simulink model "read_acs712"  (R2021b)
settings: Solver=ode1  StartTime=0.0  StopTime=30  FixedStep=0.01  RelTol=1e-3  EnableMultiTasking=on
libraries: arduinolib x3, dspstat3 x1
settings Model: ExtModeTrigDuration=2  Creator=ASUS  LastModifiedBy=ASUS
settings OptimizationCC: EnhancedBackFolding=on  PassReuseOutputArgsAs=Individual arguments  ZeroExternalMemoryAtStartup=off  ZeroInternalMemoryAtStartup=off  MaxStackSize=64  OptimizeBlockOrder=speed  DifferentSizesBufferReuse=on  OptimizationCustomize=off  EfficientTunableParamExpr=on
settings DebuggingCC: ParameterTunabilityLossMsg=error
settings HardwareCC: ProdBitPerInt=16  ProdBitPerPointer=16  ProdBitPerSizeT=16  ProdBitPerPtrDiffT=16  ProdLargestAtomicFloat=None  ProdWordSize=8  ProdHWDeviceType=Atmel->AVR
settings SFSimCC: MATLABDynamicMemAlloc=off
settings RTWCC: Description=Embedded Coder  SystemTargetFile=ert.tlc  HardwareBoard=Arduino Uno  TemplateMakefile=ert_default_tmf  Toolchain=Arduino AVR  BuildConfiguration=Faster Runs
settings CodeAppCC: ForceParamTrailComments=on  IgnoreCustomStorageClasses=off  OperatorAnnotations=on  SimulinkDataObjDesc=on  SFDataObjDesc=on  InsertBlockDesc=on
settings ERTTargetCC: SupportContinuousTime=on  SupportNonInlinedSFcns=on  SupportVariableSizeSignals=on  ExtModeTransport=3  ExtModeStaticAlloc=on  ExtModeStaticAllocSize=250  ExtModeMexFile=ext_xcp  ExtModeIntrfLevel=Level2 - Open

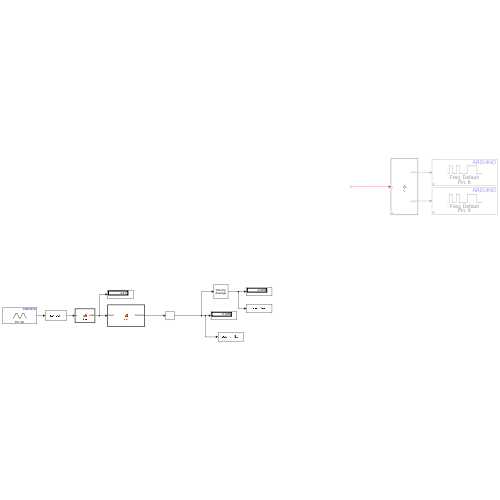
[thumbnail: Simulink's stored preview of the top-level diagram]
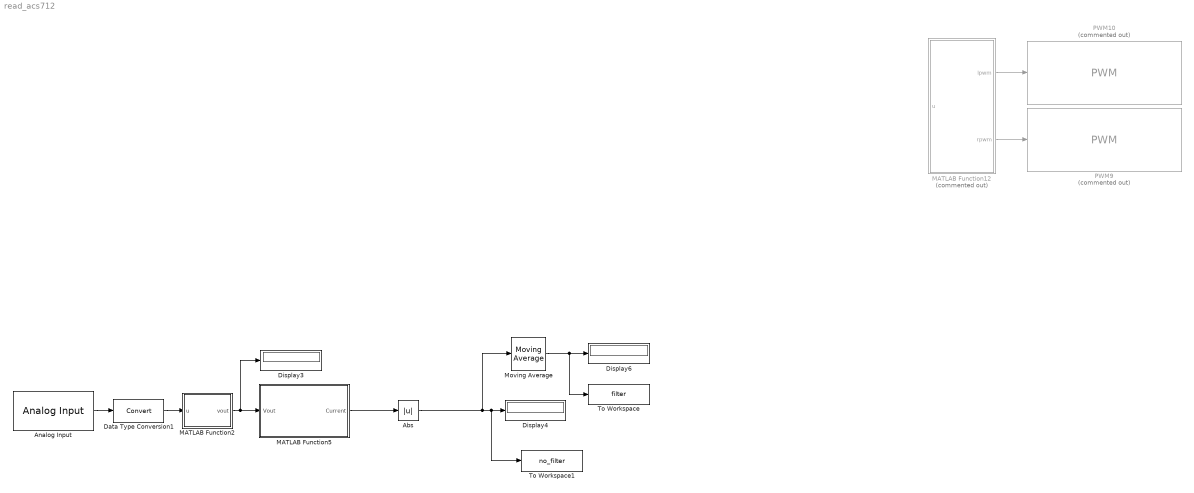
== system read_acs712 ==
  Abs : Abs
  Analog Input : arduinolib/Analog Input  pinNumber=4  ReadResultsOnly=off  ConversionTriggerSource=Software  ExternalTriggerType=uint32( 0 )  OutputDataType=uint16  EnableConversionCompleteNotify=off  EnableOuputStatus=off  SampleTime=-1  blockPlatform=arduino
  Data Type Conversion1 : DataTypeConversion
  Display3 : Display
  Display4 : Display
  Display6 : Display
  MATLAB Function12 : MATLAB Function  Commented=on  TreatAsAtomicUnit=on
  MATLAB Function2 : MATLAB Function  TreatAsAtomicUnit=on
  MATLAB Function5 : MATLAB Function  TreatAsAtomicUnit=on
  Moving Average : dspstat3/Moving Average  Method=Sliding window  ForgettingFactorPort=off  SpecifyWindowLength=on  WindowLength=100  ForgettingFactor=0.9  SimulateUsing=Code generation
  PWM10 : arduinolib/PWM  Commented=on  pinNumber=8  frequencyType=Default  desiredFrequency=490.2  achievableFrequency=490.2
  PWM9 : arduinolib/PWM  Commented=on  pinNumber=9  frequencyType=Default  desiredFrequency=490.2  achievableFrequency=490.2
  To Workspace : ToWorkspace  VariableName=filter  SampleTime=-1
  To Workspace1 : ToWorkspace  VariableName=no_filter  SampleTime=-1
  wires:
  Analog Input/1 -> Data Type Conversion1/1
  Data Type Conversion1/1 -> MATLAB Function2/1(u)
  Abs/1 -> Moving Average/1, To Workspace1/1, Display4/1
  MATLAB Function2/1(vout) -> MATLAB Function5/1(Vout), Display3/1
  Moving Average/1 -> To Workspace/1, Display6/1
  ? -> MATLAB Function12/1(u)
  MATLAB Function12/1(lpwm) -> PWM10/1
  MATLAB Function12/2(rpwm) -> PWM9/1
  MATLAB Function5/1(Current) -> Abs/1

== matlab function read_acs712/MATLAB Function5 ==
  data: Vout input; Current output
function Current = fcn(Vout)
%scale_fact = 0.185;
%zeropoint = 2.49;

scale_fact = 0.185;
zeropoint = 2.48;

Current = (Vout - zeropoint)/ scale_fact;

== matlab function read_acs712/MATLAB Function12 ==
  data: u input; lpwm output; rpwm output
function [lpwm,rpwm] = fcn(u)

Vmax = 23;
pwm = u*254/Vmax;
if pwm > 0
    lpwm = pwm;
    rpwm = 0;
elseif pwm < 0
    lpwm = 0;
    rpwm = abs(pwm);
else
    lpwm = 0;
    rpwm = 0;
end

== matlab function read_acs712/MATLAB Function2 ==
  data: u input; vout output
function vout = fcn(u)
vRef = 5;
resConv = 1024;
resADC = vRef/resConv;
vout = resADC*u;
